simulink model "StopSimulation"  (R2015b)
settings: Solver=VariableStepAuto  StartTime=0.0  StopTime=10.0  RelTol=1e-3
settings Model: Creator=LUBO  LastModifiedBy=LUBO

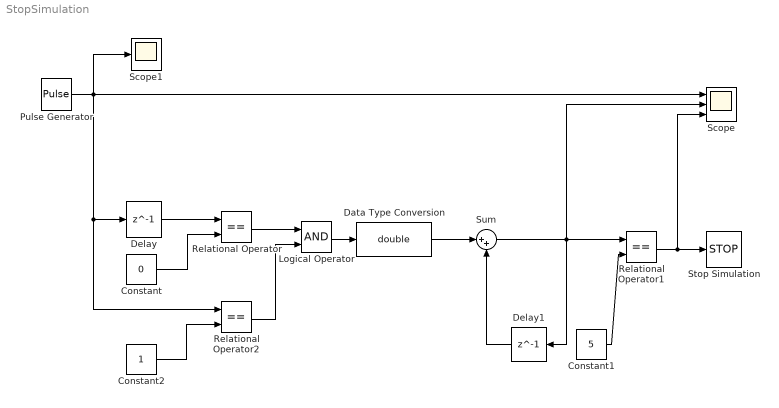
== system StopSimulation ==
  Constant : Constant  Value=0
  Constant1 : Constant  Value=5
  Constant2 : Constant
  Data Type Conversion : DataTypeConversion  OutDataTypeStr=double  LockScale=on
  Delay : Delay  DelayLength=1  InitialCondition=0  SampleTime=0.01
  Delay1 : Delay  DelayLength=1  InitialCondition=0  SampleTime=0.01
  Logical Operator : Logic  AllPortsSameDT=off  OutDataTypeStr=boolean
  Pulse Generator : DiscretePulseGenerator  PulseType=Time based  PulseWidth=50  PhaseDelay=0.2
  Relational Operator : RelationalOperator  Operator===  OutDataTypeStr=boolean
  Relational Operator1 : RelationalOperator  Operator===  OutDataTypeStr=boolean
  Relational Operator2 : RelationalOperator  Operator===  OutDataTypeStr=boolean
  Scope : Scope  NumInputPorts=3
  Scope1 : Scope
  Stop Simulation : Stop
  Sum : Sum  Inputs=|++
  wires:
  Pulse Generator/1 -> Scope1/1, Relational Operator2/1, Delay/1, Scope/1
  Relational Operator1/1 -> Scope/3, Stop Simulation/1
  Sum/1 -> Scope/2, Delay1/1, Relational Operator1/1
  Constant1/1 -> Relational Operator1/2
  Delay1/1 -> Sum/2
  Data Type Conversion/1 -> Sum/1
  Logical Operator/1 -> Data Type Conversion/1
  Relational Operator2/1 -> Logical Operator/2
  Relational Operator/1 -> Logical Operator/1
  Constant/1 -> Relational Operator/2
  Delay/1 -> Relational Operator/1
  Constant2/1 -> Relational Operator2/2
